simulink model "carma_client_test"  (Simulink 8.2)
settings: Solver=FixedStepDiscrete  SolverMode=SingleTasking  StartTime=0.0  StopTime=Inf  FixedStep=0.001  RelTol=1e-3
PostLoadFcn:
  | , if any(exist('dsrtsu_mdlpostloadfcn', 'file') == [2, 3, 6]), try dsrtsu_mdlpostloadfcn('Execute', bdroot); catch fprintf('Error in PostLoadFcn (dsrtsu_mdlpostloadfcn) for model "%s":\n %s\n', bdroot, lasterr); end, end,
libraries: carma_platform x3, rtiethernetudplib x1, parse_utils x1, srx_platform x1
settings Model: DSRTSU_INTERNAL_RTI_VER=440  DSRTSU_INTERNAL_RTI_TYPE=rti1401  DSRTSU_INTERNAL_RTIFPGA=30  Creator=leidos  LastModifiedBy=leidos  BufferReuse=off
settings DataIOCC: SignalLoggingSaveFormat=Dataset
settings OptimizationCC: BlockReduction=off  OptimizeBlockIOStorage=off  BufferReuse=off  ExpressionFolding=off  ExpressionDepthLimit=128  LocalBlockOutputs=off
settings DebuggingCC: FcnCallInpInsideContextMsg=EnableAllAsError  StateNameClashWarn=none
settings HardwareCC: ProdIntDivRoundTo=Zero  ProdEndianess=BigEndian  ProdHWDeviceType=Generic->Custom  TargetIntDivRoundTo=Zero  TargetEndianess=BigEndian  TargetHWDeviceType=Generic->Custom
settings RTWCC: SystemTargetFile=rti1401.tlc  MakeCommand=make_rti  TemplateMakefile=rti1401.tmf  Description=dSPACE DS1401 Hardware Platform  ProcessScript=rti1401_make_rtw_hook  RTWUseSimCustomCode=on
settings STFCustomTargetCC: CodeReplacementLibrary=ANSI_C  ParMdlRefBuildCompliant=on  GeneratePreprocessorConditionals=Disable all  SystemTargetFile=rti1401.tlc
settings GRTTargetCC: CompOptLevelCompliant=off  ConcurrentExecutionCompliant=off  MatFileLogging=off  ExtModeMexFile=noextcomm
settings CustomProperty: DataType=RTWOptions_EnumType_C__Program Files_dSPACE RCPHIL 2014-A_MATLAB_RTI_RTI1401_TLC_rti1401_1InitialSimState  Value=RUN
settings EnumStrPairs: String=RUN

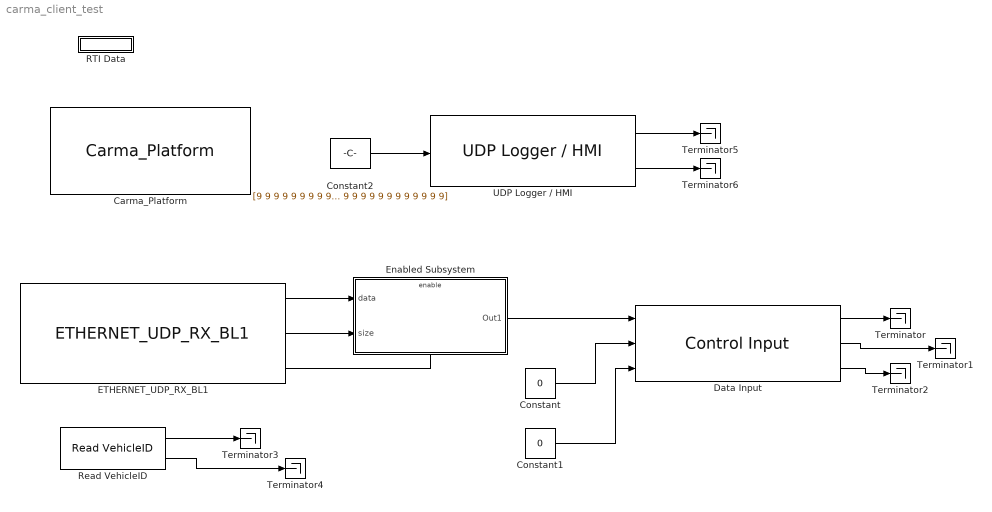
== system carma_client_test ==
  "Carma_Platform " : carma_platform/Carma_Platform 
  Constant : Constant  Value=0  OutDataTypeStr=Bus: LightCommandBus
  Constant1 : Constant  Value=0  OutDataTypeStr=Bus: LightCommandBus
  Constant2 : Constant  Value=[9 9 9 9 9 9 9 9 9 9 9 9 9 9 9 9 9 9 9 9 9 9 9 9 9 9 9 9 9 9 9 9 9 9 9 9 9 9 9 9 9 9 9 9 9 9 9 9 9 9 9 9 9 9 9 9 9 9 9 9 9 9 9 9 9 9 9 9 9 9 9 9 9 9]  OutDataTypeStr=double
  Data Input : carma_platform/Control Input
  ETHERNET_UDP_RX_BL1 : rtiethernetudplib/ETHERNET_UDP_RX_BL1  InterfaceName=rti_ethernet_interface_name  BoardType=ETH Type 1  ModuleNo=1  ChannelNo=1  SocketNo=4  MaxMessageSize=625  LocalSocket=192.168.88.21:5003  RemoteSocket=192.168.88.10:5003  DSProperties=struct('RTI',struct('Version',uint32(1),'BlockType',struct('isSLSource',uint8(1),'isSLSink',uint8(0),'isHWSource',uint8(0),'isHWSink',uint8(1),'isSetup',uint8(0),'isInline',uint8(1),'isNonInline',uint8(1),'isInterrupt',uint8(0),'isChannelwise',uint8(1)),'IOBoardType','DSETHERNETUDP','UnitType','ETHUDP','Identifier','RX','DialogType','SL','BlockSet','RTIETHERNETUDP','SlaveProcessor','NONE'))  RTIBlockInterface=struct('OutputPortsWidth',int32([1 1 1]),'OutputPortsActive',[1 1 1],'OutputPortsName',{{'Data',['Message Size'],'Status'}},'OutputPortsDataType',{{'SS_UINT32','SS_INT32','SS_BOOLEAN'}},'BlockDisplay',{{['Ethernet UDP Receive\nBoard Type: ETH Type 1\nModule: 1\nSocket: 4\nMaximum Message Size: 625'],'center'}},'IconTransparency','on','InitLevel',3,'BlockName',struct('Token',{{'ETHERNET_UDP_RX_BL1'}}),'MaskDescription',['To receive messages from the Ethernet UDP interface.'])  RTIBlockParameters=struct('InterfaceName',{{'rti_ethernet_interface_name','OFF',[]}},'BoardType',{{1,'OFF',[]}},'ModuleNo',{{1,'OFF',[1 16]}},'ChannelNo',{{1,'OFF',[1 2]}},'SocketNo',{{4,'OFF',[1 4]}},'MaxMessageSize',{{625,'ON',[1 1472]}},'LocalSocket',{{'192.168.88.21:5003','OFF',[]}},'RemoteSocket',{{'192.168.88.10:5003','OFF',[]}})  RTISFcnParameters=struct('InterfaceName','char','BoardType','double','ModuleNo','double','ChannelNo','double','SocketNo','double','MaxMessageSize','double','LocalSocket','char','RemoteSocket','char')  RTIBlockParaDefault=struct('InterfaceName','rti_ethernet_interface_name','BoardType',1,'ModuleNo',1,'ChannelNo',1,'SocketNo',1,'MaxMessageSize',625,'LocalSocket','XXX.XXX.XXX.XXX:5000','RemoteSocket','XXX.XXX.XXX.XXX:5000')
  Enabled Subsystem : Subsystem  TreatAsAtomicUnit=on
  RTI Data : Subsystem  Tag=struct('RTIDataServer',struct('RTIDataServerVs','2','RTIModelDescription','struct(''main'',''carma_client_test'',''sub'',''carma_client_test'',''isMp'',0)'))  LoadFcn="if exist('rtidc'), try,  rtidc('DataHostBlockClbLoad', gcbh); catch, disp(['Warning: ''LoadFcn'' for RTI Data block failed: ' lasterr]); end, end,"  mask(RTI_DATA_HOST){}
      mask help:
      | RTI Data Block.
      | This block is used by RTI to store internal model-dependent data.
      | Please keep this block on the root level of the model. Deleting this block will result in data loss.
      |
      | NEVER DELETE OR COPY THIS BLOCK!
      settings: CopyFcn="if exist('rtidc'), try,  rtidc('DataHostBlockClbCopy', gcbh); catch, disp(['Warning: ''CopyFcn'' for RTI Data block failed: ' lasterr]); end, end,"  DeleteFcn="if exist('rtidc'), try,  rtidc('DataHostBlockClbDelete', gcbh); catch, disp(['Warning: ''DeleteFcn'' for RTI Data block failed: ' lasterr]); end, end,"  ModelCloseFcn="if exist('rtidc'), try,  rtidc('DataHostBlockClbModelClose', gcbh); catch, disp(['Warning: ''ModelCloseFcn'' for RTI Data block failed: ' lasterr]); end, end,"  PreSaveFcn="if exist('rtidc'), try,  rtidc('DataHostBlockClbPreSave', gcbh); catch, disp(['Warning: ''PreSaveFcn'' for RTI Data block failed: ' lasterr]); end, end,"  PostSaveFcn="if exist('rtidc'), try,  rtidc('DataHostBlockClbPostSave', gcbh); catch, disp(['Warning: ''PostSaveFcn'' for RTI Data block failed: ' lasterr]); end, end,"  NameChangeFcn="if exist('rtidc'), try,  rtidc('DataHostBlockClbNameChange', gcbh); catch, disp(['Warning: ''NameChangeFcn'' for RTI Data block failed: ' lasterr]); end, end,"
      mask Help:
      | RTI Data Block.
      | This block is used by RTI to store internal model-dependent data.
      | Please keep this block on the root level of the model. Deleting this block will result in data loss.
      | 
      | NEVER DELETE OR COPY THIS BLOCK!
      mask Display:
      | text(0.5, 0.5, 'RTI Data', 'HorizontalAlignment', 'center');
      | plot([1 0]);
  Read VehicleID : srx_platform/Read VehicleID
  Terminator{,1..6} (7 alike) : Terminator
  UDP Logger / HMI : carma_platform/UDP Logger // HMI  Value=0.05
  wires:
  ETHERNET_UDP_RX_BL1/1 -> Enabled Subsystem/1("data ")
  ETHERNET_UDP_RX_BL1/2 -> Enabled Subsystem/2(size)
  ETHERNET_UDP_RX_BL1/3 -> Enabled Subsystem/Enable
  Enabled Subsystem/1(Out1) -> Data Input/1
  Data Input/1 -> Terminator/1
  Data Input/3 -> Terminator2/1
  Data Input/2 -> Terminator1/1
  Constant/1 -> Data Input/2
  Constant1/1 -> Data Input/3
  Read VehicleID/2 -> Terminator4/1
  Read VehicleID/1 -> Terminator3/1
  Constant2/1 -> UDP Logger / HMI/1
  UDP Logger / HMI/1 -> Terminator5/1
  UDP Logger / HMI/2 -> Terminator6/1

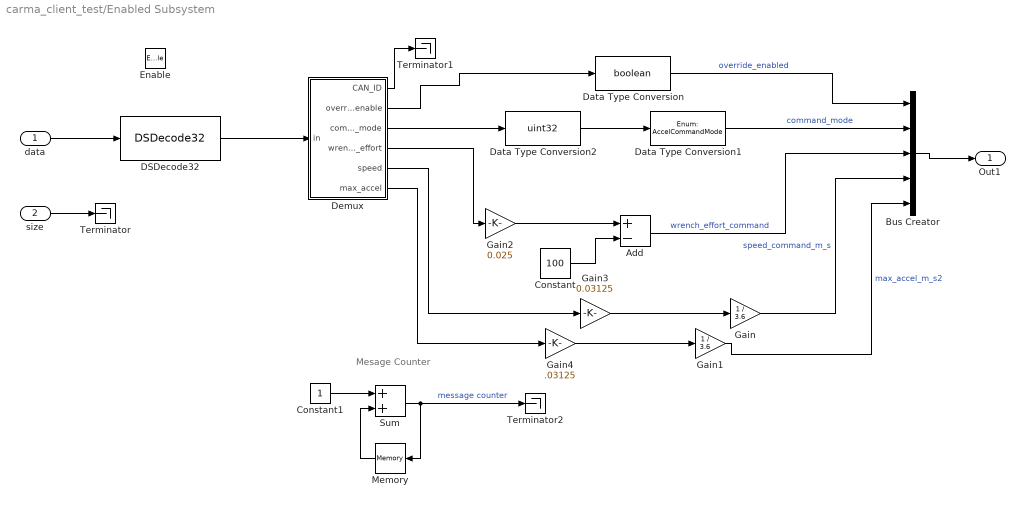
== system carma_client_test/Enabled Subsystem ==
  note: Mesage Counter
  "data " : Inport
  size : Inport  Port=2
  Enable : EnablePort
  Add : Sum  Inputs=+-
  Bus Creator : BusCreator  Inputs=5  OutDataTypeStr=Bus: AccelCommandBus
  Constant : Constant  Value=100
  Constant1 : Constant
  "DSDecode32 " : parse_utils/DSDecode32   byteordering=little endian (Intel)  offset=[0]  auto_offset=on  datatype=[5 3 3 5 5 5]  one_datatype=off  sampletime=-1
  Data Type Conversion : DataTypeConversion  OutDataTypeStr=boolean
  Data Type Conversion1 : DataTypeConversion  OutDataTypeStr=Enum: AccelCommandMode
  Data Type Conversion2 : DataTypeConversion  OutDataTypeStr=uint32
  Demux : Subsystem
  Gain : Gain  Gain=1 / 3.6
  Gain1 : Gain  Gain=1 / 3.6
  Gain2 : Gain  Gain=0.025
  Gain3 : Gain  Gain=0.03125
  Gain4 : Gain  Gain=.03125
  Memory : Memory  InheritSampleTime=on
  Sum : Sum  SaturateOnIntegerOverflow=on  InputSameDT=on  OutDataTypeStr=Inherit: Same as first input
  Terminator : Terminator
  Terminator1 : Terminator
  Terminator2 : Terminator
  Out1 : Outport
  wires:
  "data "/1 -> "DSDecode32 "/1
  "DSDecode32 "/1 -> Demux/1(in)
  size/1 -> Terminator/1
  Bus Creator/1 -> Out1/1
  Demux/1(CAN_ID) -> Terminator1/1
  Demux/5(speed) -> Gain3/1
  Demux/6(max_accel) -> Gain4/1
  Demux/3(command_mode) -> Data Type Conversion2/1
  Demux/2(override_enable) -> Data Type Conversion/1
  Data Type Conversion/1 -> Bus Creator/1  "override_enabled"
  Data Type Conversion1/1 -> Bus Creator/2  "command_mode"
  Data Type Conversion2/1 -> Data Type Conversion1/1
  Sum/1 -> Terminator2/1, Memory/1  "message counter"
  Memory/1 -> Sum/2
  Constant1/1 -> Sum/1
  Demux/4(wrench_effort) -> Gain2/1
  Gain1/1 -> Bus Creator/5  "max_accel_m_s2"
  Gain/1 -> Bus Creator/4  "speed_command_m_s"
  Gain2/1 -> Add/1
  Add/1 -> Bus Creator/3  "wrench_effort_command"
  Constant/1 -> Add/2
  Gain4/1 -> Gain1/1
  Gain3/1 -> Gain/1

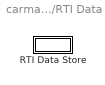
== system carma_client_test/RTI Data ==
  RTI Data Store : Subsystem  Tag=struct('private',struct('version',struct('dsVer',uint32(2)),'access',struct('modified',['26-Aug-2015 16:29:09'],'type','Model','isPerm',1)))  mask(RTI_DATA_STORE){}
      mask help:
      | RTI Data Store Block. This block is used by RTI to store internal model dependent data. Deleting this block will result in data loss.
      |
      | NEVER DELETE, COPY, OR MODIFY THIS BLOCK!
      mask Help:
      | RTI Data Store Block. This block is used by RTI to store internal model dependent data. Deleting this block will result in data loss.
      | 
      | NEVER DELETE, COPY, OR MODIFY THIS BLOCK!
      mask Display: text(0.5, 0.5, ' ', 'HorizontalAlignment', 'center');

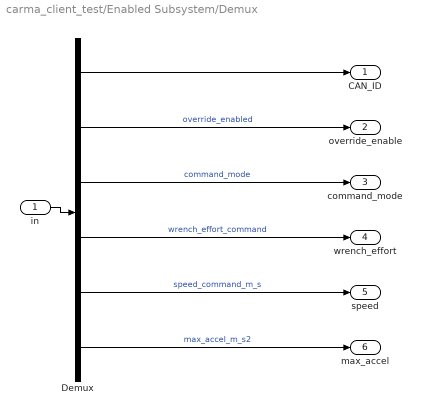
== system carma_client_test/Enabled Subsystem/Demux ==
  in : Inport
  Demux : Demux  Outputs=6
  CAN_ID : Outport
  override_enable : Outport  Port=2
  command_mode : Outport  Port=3
  wrench_effort : Outport  Port=4
  speed : Outport  Port=5
  max_accel : Outport  Port=6
  wires:
  in/1 -> Demux/1
  Demux/3 -> command_mode/1  "command_mode"
  Demux/4 -> wrench_effort/1  "wrench_effort_command"
  Demux/5 -> speed/1  "speed_command_m_s"
  Demux/6 -> max_accel/1  "max_accel_m_s2"
  Demux/1 -> CAN_ID/1
  Demux/2 -> override_enable/1  "override_enabled"

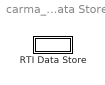
== system carma_client_test/RTI Data/RTI Data Store ==
  RTI Data Store : Subsystem  mask(RTI_DATA_STORE){}
      mask help:
      | RTI Data Store Block. This block is used by RTI to store internal model dependent data. Deleting this block will result in data loss.
      |
      | NEVER DELETE, COPY, OR MODIFY THIS BLOCK!
      mask Help:
      | RTI Data Store Block. This block is used by RTI to store internal model dependent data. Deleting this block will result in data loss.
      | 
      | NEVER DELETE, COPY, OR MODIFY THIS BLOCK!
      mask Display: text(0.5, 0.5, ' ', 'HorizontalAlignment', 'center');

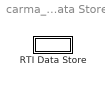
== system carma_client_test/RTI Data/RTI Data Store/RTI Data Store ==
  RTI Data Store : Subsystem  mask(RTI_DATA_STORE){}
      mask help:
      | RTI Data Store Block. This block is used by RTI to store internal model dependent data. Deleting this block will result in data loss.
      |
      | NEVER DELETE, COPY, OR MODIFY THIS BLOCK!
      mask Help:
      | RTI Data Store Block. This block is used by RTI to store internal model dependent data. Deleting this block will result in data loss.
      | 
      | NEVER DELETE, COPY, OR MODIFY THIS BLOCK!
      mask Display: text(0.5, 0.5, ' ', 'HorizontalAlignment', 'center');

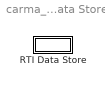
== system carma_client_test/RTI Data/RTI Data Store/RTI Data Store/RTI Data Store ==
  RTI Data Store : Subsystem  mask(RTI_DATA_STORE){}
      mask help:
      | RTI Data Store Block. This block is used by RTI to store internal model dependent data. Deleting this block will result in data loss.
      |
      | NEVER DELETE, COPY, OR MODIFY THIS BLOCK!
      mask Help:
      | RTI Data Store Block. This block is used by RTI to store internal model dependent data. Deleting this block will result in data loss.
      | 
      | NEVER DELETE, COPY, OR MODIFY THIS BLOCK!
      mask Display: text(0.5, 0.5, ' ', 'HorizontalAlignment', 'center');

== system carma_client_test/RTI Data/RTI Data Store/RTI Data Store/RTI Data Store/RTI Data Store ==
